simulink model "PubIfStateAEB_MDL"  (R2020b)
settings: configuration reference "DspaceConfig" (kept outside this file)
PostLoadFcn:
  | if any(exist('dsrtsu_mdlpostloadfcn', 'file') ~= 0), dsrtsu_mdlpostloadfcn('Execute', bdroot); end
InitFcn:
  | , if any(exist('dsmpb_private', 'file') ~= 0), dsmpb_private('dsmpb_mdlclblib', 'Init', bdroot); end,
PreSaveFcn:
  | , if any(exist('dsmpb_private', 'file') ~= 0), dsmpb_private('dsmpb_mdlclblib', 'PreSave', bdroot); end,
CloseFcn:
  | , if any(exist('dsmpb_private', 'file') ~= 0), dsmpb_private('dsmpb_mdlclblib', 'Close', bdroot); end,
settings Model: DataDictionary=HWA_DDs.sldd  RTICANMMDATA=struct('GeneralSetupData',struct('modelroot','C:\Users\GW00133806\Desktop\ADAS_Store\Project\V61_Autobox_Noa_Nofusion\Com','generalsettings',struct('filesettings',struct('destfolder',struct('Name','RTICANMM_FILES','Check',1),'buildfolder',struct('Name','.','Check',1),'AbsDestfolder',struct('Name','C:\Users\GW00133806\Desktop\ADAS_Store\Project\V61_Autobox_Noa_Nofusion\Com\RTICANMM_FILES'),'AbsBuildfolder',struct('Name','C:\Users\GW00133806\Desktop\ADAS_Store\Project\V61_Autobox_Noa_Nofusion\Com'))),'options',struct('addpaths',1,'rmpaths',1,'addtrcexclusion',false,'cannavigator',struct('checkmonitoring',0),'show_usrtrc',0,'use_usrtrc',0),'advanced',struct('options',ones(1,100)),'MPSetup',{{}},'RTI',struct('Type','DSRT','Ver','4.2','Date','02-Nov-2019'),'modelname','PubIfStateAEB_MDL','block','PubIfStateAEB_MDL'))  DSRTSU_INTERNAL_RTIFPGA=150  Creator=GW00180895  LastModifiedBy=GW00133806
settings ConfigSetRef: SourceName=DspaceConfig

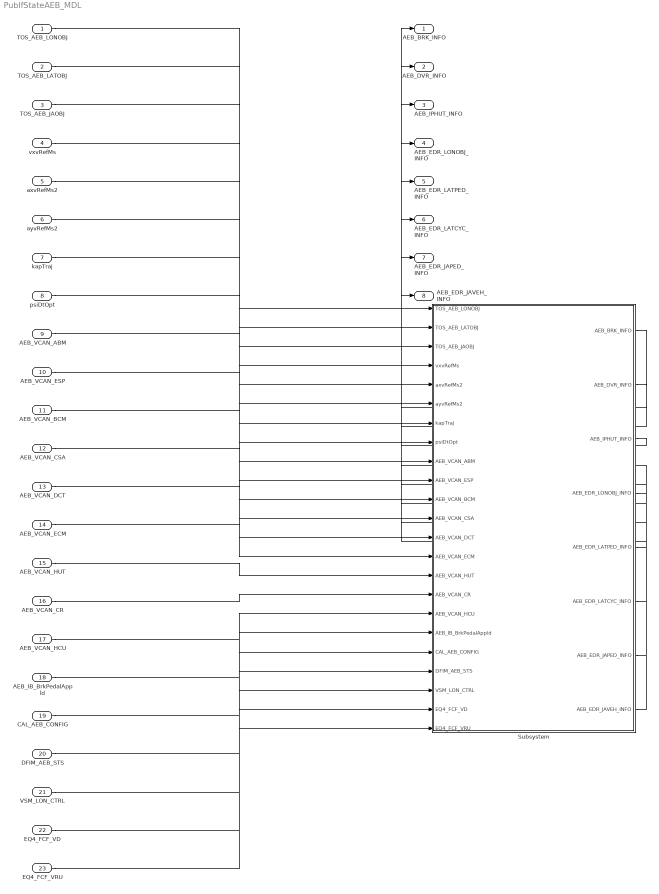
== system PubIfStateAEB_MDL ==
  TOS_AEB_LONOBJ : Inport  OutDataTypeStr=Bus: TOS_AEB_LONOBJ_BUS  PortDimensions=1  BusOutputAsStruct=on
  TOS_AEB_LATOBJ : Inport  Port=2  OutDataTypeStr=Bus: TOS_AEB_LATOBJ_BUS  PortDimensions=10  BusOutputAsStruct=on
  TOS_AEB_JAOBJ : Inport  Port=3  OutDataTypeStr=Bus: TOS_AEB_JAOBJ_BUS  PortDimensions=32  BusOutputAsStruct=on
  vxvRefMs : Inport  Port=4  OutDataTypeStr=single  PortDimensions=1  BusOutputAsStruct=on
  axvRefMs2 : Inport  Port=5  OutDataTypeStr=single  PortDimensions=1  BusOutputAsStruct=on
  ayvRefMs2 : Inport  Port=6  OutDataTypeStr=single  PortDimensions=1  BusOutputAsStruct=on
  kapTraj : Inport  Port=7  OutDataTypeStr=single  PortDimensions=1  BusOutputAsStruct=on
  psiDtOpt : Inport  Port=8  OutDataTypeStr=single  PortDimensions=1  BusOutputAsStruct=on
  AEB_VCAN_ABM : Inport  Port=9  OutDataTypeStr=Bus: AEB_VCAN_ABM_BUS  PortDimensions=1  BusOutputAsStruct=on
  AEB_VCAN_ESP : Inport  Port=10  OutDataTypeStr=Bus: AEB_VCAN_ESP_BUS  PortDimensions=1  BusOutputAsStruct=on
  AEB_VCAN_BCM : Inport  Port=11  OutDataTypeStr=Bus: AEB_VCAN_BCM_BUS  PortDimensions=1  BusOutputAsStruct=on
  AEB_VCAN_CSA : Inport  Port=12  OutDataTypeStr=Bus: AEB_VCAN_CSA_BUS  PortDimensions=1  BusOutputAsStruct=on
  AEB_VCAN_DCT : Inport  Port=13  OutDataTypeStr=Bus: AEB_VCAN_DCT_BUS  PortDimensions=1  BusOutputAsStruct=on
  AEB_VCAN_ECM : Inport  Port=14  OutDataTypeStr=Bus: AEB_VCAN_ECM_BUS  PortDimensions=1  BusOutputAsStruct=on
  AEB_VCAN_HUT : Inport  Port=15  OutDataTypeStr=Bus: AEB_VCAN_HUT_BUS  PortDimensions=1  BusOutputAsStruct=on
  AEB_VCAN_CR : Inport  Port=16  OutDataTypeStr=Bus: AEB_VCAN_CR_BUS  PortDimensions=1  BusOutputAsStruct=on
  AEB_VCAN_HCU : Inport  Port=17  OutDataTypeStr=Bus: AEB_VCAN_HCU_BUS  PortDimensions=1  BusOutputAsStruct=on
  AEB_IB_BrkPedalAppld : Inport  Port=18  OutDataTypeStr=boolean  PortDimensions=1  BusOutputAsStruct=on
  CAL_AEB_CONFIG : Inport  Port=19  OutDataTypeStr=Bus: CAL_AEB_CONFIG_BUS  PortDimensions=1  BusOutputAsStruct=on
  DFIM_AEB_STS : Inport  Port=20  OutDataTypeStr=Bus: DFIM_AEB_STS_BUS  PortDimensions=1  BusOutputAsStruct=on
  VSM_LON_CTRL : Inport  Port=21  OutDataTypeStr=Bus: VSM_LON_CTRL_BUS  PortDimensions=1  BusOutputAsStruct=on
  EQ4_FCF_VD : Inport  Port=22  OutDataTypeStr=Bus: EQ4_FCF_VD_BUS  PortDimensions=1  BusOutputAsStruct=on
  EQ4_FCF_VRU : Inport  Port=23  OutDataTypeStr=Bus: EQ4_FCF_VRU_BUS  PortDimensions=1  BusOutputAsStruct=on
  Subsystem : Subsystem
  AEB_BRK_INFO : Outport  OutDataTypeStr=Bus: AEB_BRK_INFO_BUS  PortDimensions=1  BusOutputAsStruct=on
  AEB_DVR_INFO : Outport  Port=2  OutDataTypeStr=Bus: AEB_DVR_INFO_BUS  PortDimensions=1  BusOutputAsStruct=on
  AEB_IPHUT_INFO : Outport  Port=3  OutDataTypeStr=Bus: AEB_IPHUT_INFO_BUS  PortDimensions=1  BusOutputAsStruct=on
  AEB_EDR_LONOBJ_INFO : Outport  Port=4  OutDataTypeStr=Bus: AEB_EDR_LONOBJ_INFO_BUS  PortDimensions=1  BusOutputAsStruct=on
  AEB_EDR_LATPED_INFO : Outport  Port=5  OutDataTypeStr=Bus: AEB_EDR_LATPED_INFO_BUS  PortDimensions=1  BusOutputAsStruct=on
  AEB_EDR_LATCYC_INFO : Outport  Port=6  OutDataTypeStr=Bus: AEB_EDR_LATCYC_INFO_BUS  PortDimensions=1  BusOutputAsStruct=on
  AEB_EDR_JAPED_INFO : Outport  Port=7  OutDataTypeStr=Bus: AEB_EDR_JAPED_INFO_BUS  PortDimensions=1  BusOutputAsStruct=on
  AEB_EDR_JAVEH_INFO : Outport  Port=8  OutDataTypeStr=Bus: AEB_EDR_JAVEH_INFO_BUS  PortDimensions=1  BusOutputAsStruct=on
  wires:
  TOS_AEB_LONOBJ/1 -> Subsystem/1(TOS_AEB_LONOBJ)
  TOS_AEB_LATOBJ/1 -> Subsystem/2(TOS_AEB_LATOBJ)
  TOS_AEB_JAOBJ/1 -> Subsystem/3(TOS_AEB_JAOBJ)
  vxvRefMs/1 -> Subsystem/4(vxvRefMs)
  axvRefMs2/1 -> Subsystem/5(axvRefMs2)
  ayvRefMs2/1 -> Subsystem/6(ayvRefMs2)
  kapTraj/1 -> Subsystem/7(kapTraj)
  psiDtOpt/1 -> Subsystem/8(psiDtOpt)
  AEB_VCAN_ABM/1 -> Subsystem/9(AEB_VCAN_ABM)
  AEB_VCAN_ESP/1 -> Subsystem/10(AEB_VCAN_ESP)
  AEB_VCAN_BCM/1 -> Subsystem/11(AEB_VCAN_BCM)
  AEB_VCAN_CSA/1 -> Subsystem/12(AEB_VCAN_CSA)
  AEB_VCAN_DCT/1 -> Subsystem/13(AEB_VCAN_DCT)
  AEB_VCAN_ECM/1 -> Subsystem/14(AEB_VCAN_ECM)
  AEB_VCAN_HUT/1 -> Subsystem/15(AEB_VCAN_HUT)
  AEB_VCAN_CR/1 -> Subsystem/16(AEB_VCAN_CR)
  AEB_VCAN_HCU/1 -> Subsystem/17(AEB_VCAN_HCU)
  AEB_IB_BrkPedalAppld/1 -> Subsystem/18(AEB_IB_BrkPedalAppld)
  CAL_AEB_CONFIG/1 -> Subsystem/19(CAL_AEB_CONFIG)
  DFIM_AEB_STS/1 -> Subsystem/20(DFIM_AEB_STS)
  VSM_LON_CTRL/1 -> Subsystem/21(VSM_LON_CTRL)
  EQ4_FCF_VD/1 -> Subsystem/22(EQ4_FCF_VD)
  EQ4_FCF_VRU/1 -> Subsystem/23(EQ4_FCF_VRU)
  Subsystem/1(AEB_BRK_INFO) -> AEB_BRK_INFO/1
  Subsystem/2(AEB_DVR_INFO) -> AEB_DVR_INFO/1
  Subsystem/3(AEB_IPHUT_INFO) -> AEB_IPHUT_INFO/1
  Subsystem/4(AEB_EDR_LONOBJ_INFO) -> AEB_EDR_LONOBJ_INFO/1
  Subsystem/5(AEB_EDR_LATPED_INFO) -> AEB_EDR_LATPED_INFO/1
  Subsystem/6(AEB_EDR_LATCYC_INFO) -> AEB_EDR_LATCYC_INFO/1
  Subsystem/7(AEB_EDR_JAPED_INFO) -> AEB_EDR_JAPED_INFO/1
  Subsystem/8(AEB_EDR_JAVEH_INFO) -> AEB_EDR_JAVEH_INFO/1

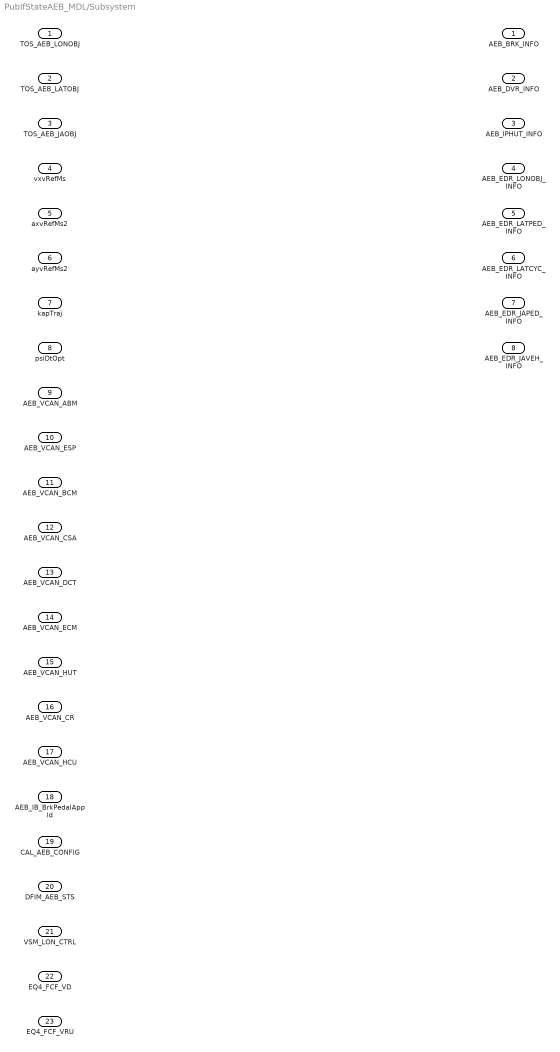
== system PubIfStateAEB_MDL/Subsystem ==
  TOS_AEB_LONOBJ : Inport  OutDataTypeStr=Bus: TOS_AEB_LONOBJ_BUS  PortDimensions=1  BusOutputAsStruct=on
  TOS_AEB_LATOBJ : Inport  Port=2  OutDataTypeStr=Bus: TOS_AEB_LATOBJ_BUS  PortDimensions=10  BusOutputAsStruct=on
  TOS_AEB_JAOBJ : Inport  Port=3  OutDataTypeStr=Bus: TOS_AEB_JAOBJ_BUS  PortDimensions=32  BusOutputAsStruct=on
  vxvRefMs : Inport  Port=4  OutDataTypeStr=single  PortDimensions=1  BusOutputAsStruct=on
  axvRefMs2 : Inport  Port=5  OutDataTypeStr=single  PortDimensions=1  BusOutputAsStruct=on
  ayvRefMs2 : Inport  Port=6  OutDataTypeStr=single  PortDimensions=1  BusOutputAsStruct=on
  kapTraj : Inport  Port=7  OutDataTypeStr=single  PortDimensions=1  BusOutputAsStruct=on
  psiDtOpt : Inport  Port=8  OutDataTypeStr=single  PortDimensions=1  BusOutputAsStruct=on
  AEB_VCAN_ABM : Inport  Port=9  OutDataTypeStr=Bus: AEB_VCAN_ABM_BUS  PortDimensions=1  BusOutputAsStruct=on
  AEB_VCAN_ESP : Inport  Port=10  OutDataTypeStr=Bus: AEB_VCAN_ESP_BUS  PortDimensions=1  BusOutputAsStruct=on
  AEB_VCAN_BCM : Inport  Port=11  OutDataTypeStr=Bus: AEB_VCAN_BCM_BUS  PortDimensions=1  BusOutputAsStruct=on
  AEB_VCAN_CSA : Inport  Port=12  OutDataTypeStr=Bus: AEB_VCAN_CSA_BUS  PortDimensions=1  BusOutputAsStruct=on
  AEB_VCAN_DCT : Inport  Port=13  OutDataTypeStr=Bus: AEB_VCAN_DCT_BUS  PortDimensions=1  BusOutputAsStruct=on
  AEB_VCAN_ECM : Inport  Port=14  OutDataTypeStr=Bus: AEB_VCAN_ECM_BUS  PortDimensions=1  BusOutputAsStruct=on
  AEB_VCAN_HUT : Inport  Port=15  OutDataTypeStr=Bus: AEB_VCAN_HUT_BUS  PortDimensions=1  BusOutputAsStruct=on
  AEB_VCAN_CR : Inport  Port=16  OutDataTypeStr=Bus: AEB_VCAN_CR_BUS  PortDimensions=1  BusOutputAsStruct=on
  AEB_VCAN_HCU : Inport  Port=17  OutDataTypeStr=Bus: AEB_VCAN_HCU_BUS  PortDimensions=1  BusOutputAsStruct=on
  AEB_IB_BrkPedalAppld : Inport  Port=18  OutDataTypeStr=boolean  PortDimensions=1  BusOutputAsStruct=on
  CAL_AEB_CONFIG : Inport  Port=19  OutDataTypeStr=Bus: CAL_AEB_CONFIG_BUS  PortDimensions=1  BusOutputAsStruct=on
  DFIM_AEB_STS : Inport  Port=20  OutDataTypeStr=Bus: DFIM_AEB_STS_BUS  PortDimensions=1  BusOutputAsStruct=on
  VSM_LON_CTRL : Inport  Port=21  OutDataTypeStr=Bus: VSM_LON_CTRL_BUS  PortDimensions=1  BusOutputAsStruct=on
  EQ4_FCF_VD : Inport  Port=22  OutDataTypeStr=Bus: EQ4_FCF_VD_BUS  PortDimensions=1  BusOutputAsStruct=on
  EQ4_FCF_VRU : Inport  Port=23  OutDataTypeStr=Bus: EQ4_FCF_VRU_BUS  PortDimensions=1  BusOutputAsStruct=on
  AEB_BRK_INFO : Outport  OutDataTypeStr=Bus: AEB_BRK_INFO_BUS  PortDimensions=1  BusOutputAsStruct=on
  AEB_DVR_INFO : Outport  Port=2  OutDataTypeStr=Bus: AEB_DVR_INFO_BUS  PortDimensions=1  BusOutputAsStruct=on
  AEB_IPHUT_INFO : Outport  Port=3  OutDataTypeStr=Bus: AEB_IPHUT_INFO_BUS  PortDimensions=1  BusOutputAsStruct=on
  AEB_EDR_LONOBJ_INFO : Outport  Port=4  OutDataTypeStr=Bus: AEB_EDR_LONOBJ_INFO_BUS  PortDimensions=1  BusOutputAsStruct=on
  AEB_EDR_LATPED_INFO : Outport  Port=5  OutDataTypeStr=Bus: AEB_EDR_LATPED_INFO_BUS  PortDimensions=1  BusOutputAsStruct=on
  AEB_EDR_LATCYC_INFO : Outport  Port=6  OutDataTypeStr=Bus: AEB_EDR_LATCYC_INFO_BUS  PortDimensions=1  BusOutputAsStruct=on
  AEB_EDR_JAPED_INFO : Outport  Port=7  OutDataTypeStr=Bus: AEB_EDR_JAPED_INFO_BUS  PortDimensions=1  BusOutputAsStruct=on
  AEB_EDR_JAVEH_INFO : Outport  Port=8  OutDataTypeStr=Bus: AEB_EDR_JAVEH_INFO_BUS  PortDimensions=1  BusOutputAsStruct=on
